simulink model "Q3_HW6S"  (R2023a)
settings: Solver=VariableStepAuto  StartTime=0.0  StopTime=12  RelTol=1e-3
values from neighbouring files (symbols this model uses):
  A = [ 0 1 0;0 0 1;6 -1 -4]    [Q3_HW6.m]    (also in Q4_HW6.m = [0 1; 0 -1])
  B = [ 0 0 1]'    [Q3_HW6.m]    (also in Q4_HW6.m = [0; 1])
  C = [10 1 0]    [Q3_HW6.m]
  k = place(A,B,[-3 -1.5+2i -1.5-2i])    [Q3_HW6.m]
settings Model: Creator=Habib  LastModifiedBy=Habib

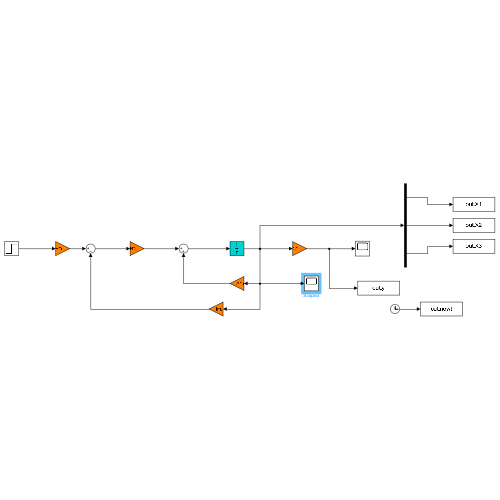
[thumbnail: Simulink's stored preview of the top-level diagram]
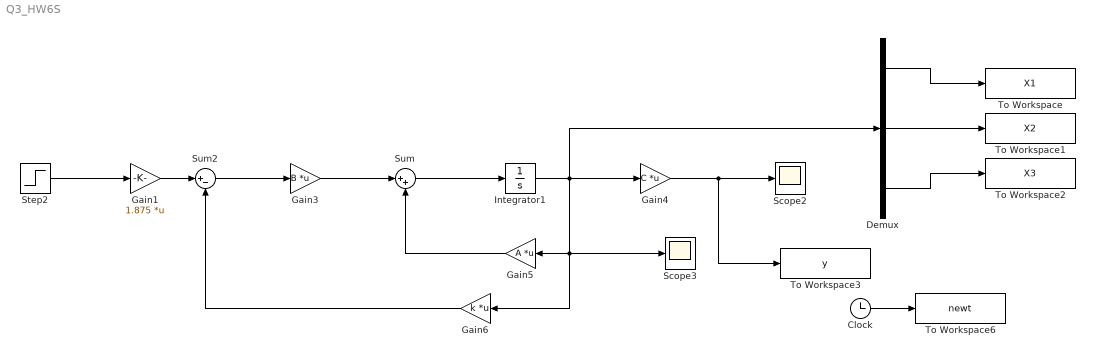
== system Q3_HW6S ==
  Clock : Clock
  Demux : Demux  Outputs=3
  Gain1 : Gain  Gain=1.875  Multiplication=Matrix(K*u)
  Gain3 : Gain  Gain=B  Multiplication=Matrix(K*u)
  Gain4 : Gain  Gain=C  Multiplication=Matrix(K*u)
  Gain5 : Gain  Gain=A  Multiplication=Matrix(K*u)
  Gain6 : Gain  Gain=k  Multiplication=Matrix(K*u)
  Integrator1 : Integrator  InitialCondition=[1 1 1]
  Scope2 : Scope
  Scope3 : Scope
  Step2 : Step  Time=0  SampleTime=0
  Sum : Sum  Inputs=|++
  Sum2 : Sum  Inputs=|+-
  To Workspace : ToWorkspace  VariableName=X1  SampleTime=-1
      settings: Save2DSignal=2-D array (concatenate along first dimension)
  To Workspace1 : ToWorkspace  VariableName=X2  SampleTime=-1
      settings: Save2DSignal=2-D array (concatenate along first dimension)
  To Workspace2 : ToWorkspace  VariableName=X3  SampleTime=-1
      settings: Save2DSignal=2-D array (concatenate along first dimension)
  To Workspace3 : ToWorkspace  VariableName=y  SampleTime=-1
  To Workspace6 : ToWorkspace  VariableName=newt  SaveFormat=Timeseries  SampleTime=-1
  wires:
  Clock/1 -> To Workspace6/1
  Gain4/1 -> To Workspace3/1, Scope2/1
  Demux/2 -> To Workspace1/1
  Demux/3 -> To Workspace2/1
  Demux/1 -> To Workspace/1
  Gain6/1 -> Sum2/2
  Sum/1 -> Integrator1/1
  Integrator1/1 -> Gain6/1, Scope3/1, Gain5/1, Demux/1, Gain4/1
  Sum2/1 -> Gain3/1
  Gain5/1 -> Sum/2
  Gain3/1 -> Sum/1
  Gain1/1 -> Sum2/1
  Step2/1 -> Gain1/1
